simulink model "Room"  (R2020b)
settings: Solver=FixedStepAuto  StartTime=0  StopTime=48  FixedStep=0.1  RelTol=1e-3
settings Model: Creator=jimd  LastModifiedBy=jimd

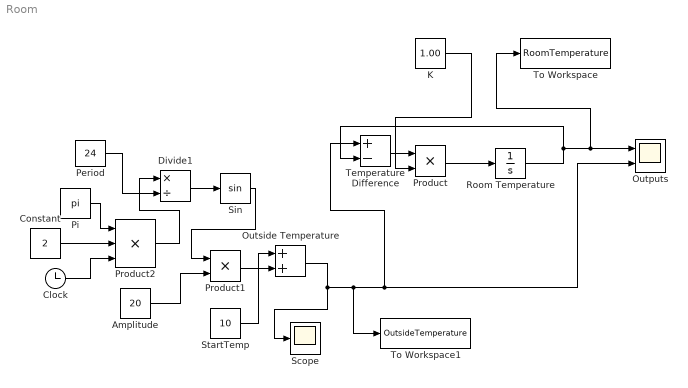
== system Room ==
  Amplitude : Constant  Value=20
  Clock : Clock
  Constant : Constant  Value=2
  Divide1 : Product  Inputs=*/
  K : Constant  Value=1.00
  Outputs : Scope  NumInputPorts=2
  Outside Temperature : Sum
  Period : Constant  Value=24
  Pi : Constant  Value=pi  OutDataTypeStr=Inherit: Inherit via back propagation
  Product : Product
  Product1 : Product
  Product2 : Product  Inputs=3
  Room Temperature : Integrator  InitialCondition=10
  Scope : Scope
  Sin : Trigonometry
  StartTemp : Constant  Value=10
  Temperature Difference : Sum  Inputs=+-
  To Workspace : ToWorkspace  VariableName=RoomTemperature  SaveFormat=Timeseries  SampleTime=-1
  To Workspace1 : ToWorkspace  VariableName=OutsideTemperature  SaveFormat=Timeseries  SampleTime=-1
  wires:
  Temperature Difference/1 -> Product/1
  K/1 -> Product/2
  Room Temperature/1 -> Temperature Difference/2, To Workspace/1, Outputs/1
  Product/1 -> Room Temperature/1
  Pi/1 -> Product2/1
  Constant/1 -> Product2/2
  Clock/1 -> Product2/3
  Product2/1 -> Divide1/1
  Period/1 -> Divide1/2
  Divide1/1 -> Sin/1
  Sin/1 -> Product1/1
  Amplitude/1 -> Product1/2
  Product1/1 -> Outside Temperature/1
  StartTemp/1 -> Outside Temperature/2
  Outside Temperature/1 -> To Workspace1/1, Temperature Difference/1, Outputs/2, Scope/1
